simulink model "DC_w_load_R2018a"  (R2018a)
settings: Solver=VariableStepAuto  StartTime=0.0  StopTime=1  MaxStep=1e-4  RelTol=1e-3
values from neighbouring files (symbols this model uses):
  gr = 1024    [DC_twin_parameters.m]
  J = 2.56e4    (= 25600)    [Apollo_LM_design_discrete_observer.m]    (also in Apollo_LM_design_observer.m; Apollo_LM_observer_feedback.m; Apollo_LM_state_feedback.m; DC_twin_parameters.m = 22.8675707733)
  k = Vnom / w_no_load    (= 0.0309706916287)    [DC_twin_parameters.m]    (also in partial_exam_facit.m = 2)
  k2 = (1+sqrt(2))*n^2/tauc^2/gM    [Apollo_LM_observer_feedback.m]
  L = place(A, B, pd)    [Apollo_LM_design_discrete_observer.m]    (also in Apollo_LM_design_observer.m = L_a; Apollo_LM_observer_feedback.m = [l1, l2, l3]; Apollo_LM_state_feedback.m = [l1, l2, l3]; DC_twin_parameters.m = 0.000268)
  R = 1.75    [DC_twin_parameters.m]
settings Model: Creator=kjartan  LastModifiedBy=kjartan
settings DataIOCC: ReturnWorkspaceOutputs=on
settings DebuggingCC: SFMachineParentedDataDiag=error
settings SFSimCC: SimUseLocalCustomCode=on
settings RTWCC: RTWUseLocalCustomCode=on

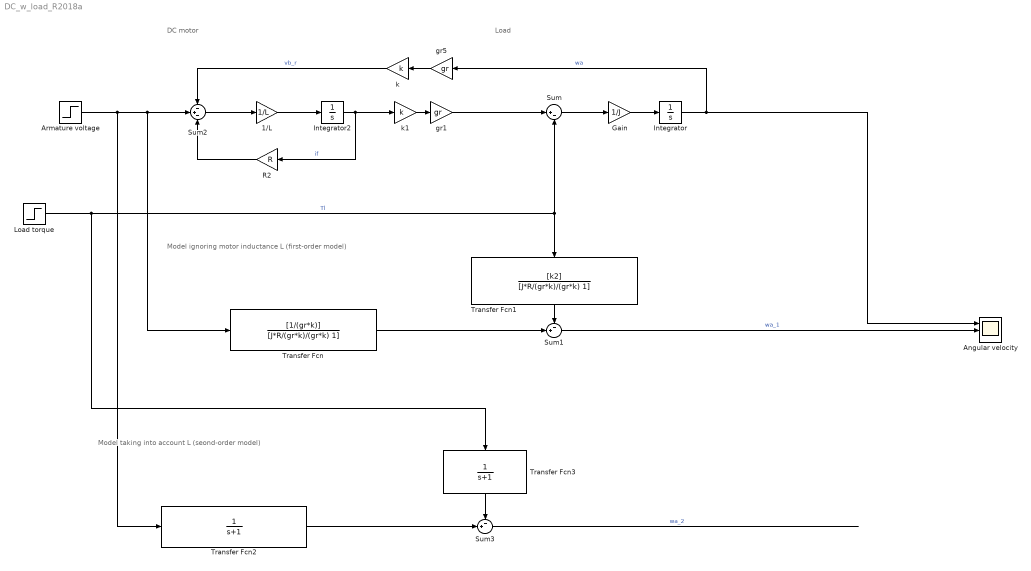
== system DC_w_load_R2018a ==
  note: Model ignoring motor inductance L (first-order model)
  note: Load
  note: DC motor
  note: Model taking into account L (seond-order model)
  1/L : Gain  Gain=1/L
  Angular velocity : Scope  NumInputPorts=3
  Armature voltage : Step  Time=0  After=12  SampleTime=0
  Gain : Gain  Gain=1/J
  Integrator : Integrator
  Integrator2 : Integrator
  Load torque : Step  Time=0.5  After=10  SampleTime=0
  R2 : Gain  Gain=R
  Sum : Sum  Inputs=|+-
  Sum1 : Sum  Inputs=-+|
  Sum2 : Sum  Inputs=-+-
  Sum3 : Sum  Inputs=-+|
  Transfer Fcn : TransferFcn  Numerator=[1/(gr*k)]  Denominator=[J*R/(gr*k)/(gr*k) 1]
  Transfer Fcn1 : TransferFcn  Numerator=[k2]  Denominator=[J*R/(gr*k)/(gr*k) 1]
  Transfer Fcn2 : TransferFcn  Denominator=[1 1]
  Transfer Fcn3 : TransferFcn  Denominator=[1 1]
  gr1 : Gain  Gain=gr
  gr5 : Gain  Gain=gr
  k : Gain  Gain=k
  k1 : Gain  Gain=k
  wires:
  gr5/1 -> k/1
  R2/1 -> Sum2/3
  Integrator2/1 -> R2/1, k1/1  "if"
  Sum2/1 -> 1/L/1
  k1/1 -> gr1/1
  1/L/1 -> Integrator2/1
  k/1 -> Sum2/1  "vb_r"
  Sum/1 -> Gain/1
  Gain/1 -> Integrator/1
  Integrator/1 -> gr5/1, Angular velocity/1  "wa"
  gr1/1 -> Sum/1
  Transfer Fcn/1 -> Sum1/2
  Transfer Fcn1/1 -> Sum1/1
  Sum1/1 -> Angular velocity/2  "wa_1"
  Sum3/1 -> ?  "wa_2"
  Transfer Fcn2/1 -> Sum3/2
  Load torque/1 -> Transfer Fcn1/1, Sum/2, Transfer Fcn3/1  "Tl"
  Transfer Fcn3/1 -> Sum3/1
  Armature voltage/1 -> Transfer Fcn2/1, Transfer Fcn/1, Sum2/2
